simulink model "GHV_open_equation"  (R2023b)
settings: Solver=VariableStepAuto  StartTime=0.0  StopTime=10  FixedStep=0.0000001  MaxStep=0.1  RelTol=1e-3
libraries: simulink_extras x2
settings Model: SimulationMode=accelerator  Creator=Admin  LastModifiedBy=Admin

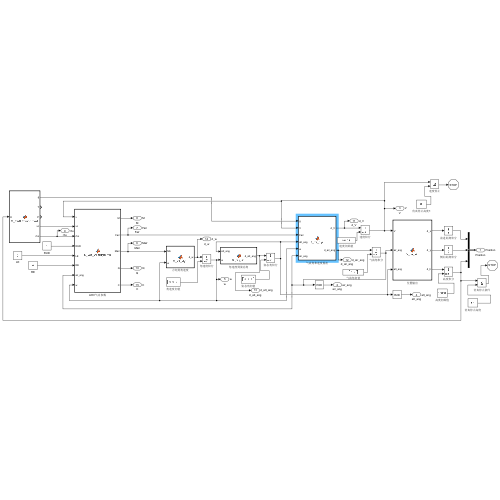
[thumbnail: Simulink's stored preview of the top-level diagram]
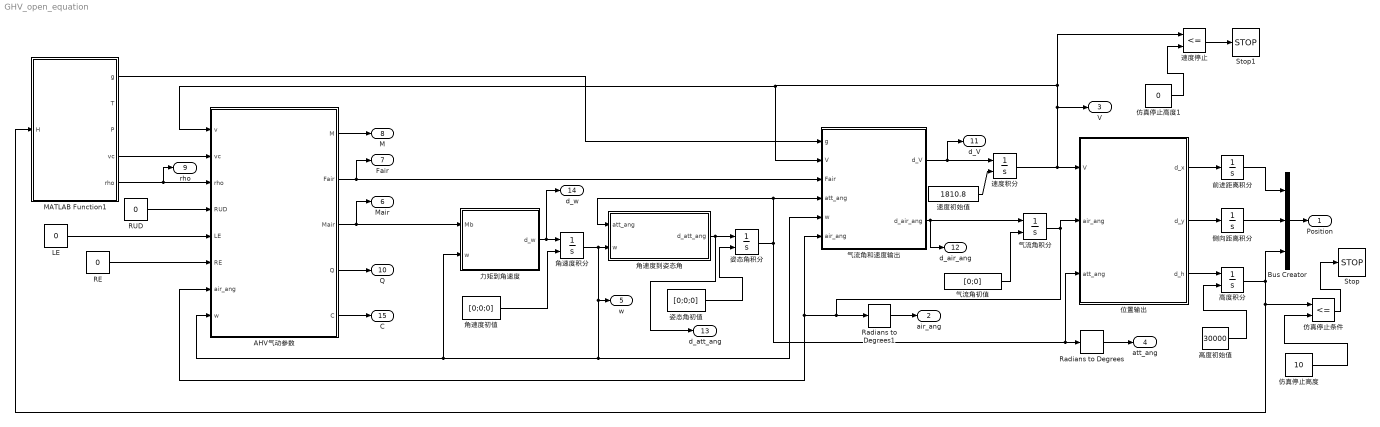
== system GHV_open_equation ==
  AHV气动参数 : MATLAB Function  TreatAsAtomicUnit=on
  Bus Creator : BusCreator  Inputs=3
  LE : Constant  Value=0
  MATLAB Function1 : MATLAB Function  TreatAsAtomicUnit=on
  RE : Constant  Value=0
  RUD : Constant  Value=0
  Radians to Degrees : simulink_extras/Transformations/Radians to Degrees
  Radians to Degrees1 : simulink_extras/Transformations/Radians to Degrees
  Stop : Stop
  Stop1 : Stop
  仿真停止条件 : RelationalOperator  Operator=<=  OutDataTypeStr=boolean  RndMeth=Simplest  InputSameDT=off
  仿真停止高度 : Constant  Value=10
  仿真停止高度1 : Constant  Value=0
  位置输出 : MATLAB Function  TreatAsAtomicUnit=on
  侧向距离积分 : Integrator
  前进距离积分 : Integrator
  力矩到角速度 : MATLAB Function  TreatAsAtomicUnit=on
  姿态角初值 : Constant  Value=[0;0;0]
  姿态角积分 : Integrator  InitialConditionSource=external  InitialCondition=[0;0;0]
  气流角初值 : Constant  Value=[0;0]
  气流角和速度输出 : MATLAB Function  TreatAsAtomicUnit=on
  气流角积分 : Integrator  InitialConditionSource=external  InitialCondition=[0;0]
  角速度初值 : Constant  Value=[0;0;0]
  角速度到姿态角 : MATLAB Function  TreatAsAtomicUnit=on
  角速度积分 : Integrator  InitialConditionSource=external  InitialCondition=[0;0;0]
  速度停止 : RelationalOperator  Operator=<=  OutDataTypeStr=boolean  RndMeth=Simplest  InputSameDT=off
  速度初始值 : Constant  Value=1810.8
  速度积分 : Integrator  InitialConditionSource=external  InitialCondition=2*340
  高度初始值 : Constant  Value=30000
  高度积分 : Integrator  InitialConditionSource=external  InitialCondition=80000
  Position : Outport  SignalName=Position
  air_ang : Outport  Port=2  SignalName=air_ang
  V : Outport  Port=3  SignalName=V
  att_ang : Outport  Port=4  SignalName=att_ang
  w : Outport  Port=5  SignalName=w
  Mair : Outport  Port=6  SignalName=Mair
  Fair : Outport  Port=7  SignalName=Fair
  M : Outport  Port=8  SignalName=M
  rho : Outport  Port=9  SignalName=rho
  Q : Outport  Port=10  SignalName=Q
  d_V : Outport  Port=11  SignalName=d_V
  d_air_ang : Outport  Port=12  SignalName=d_air_ang
  d_att_ang : Outport  Port=13  SignalName=d_att_ang
  d_w : Outport  Port=14  SignalName=d_w
  C : Outport  Port=15  SignalName=C
  wires:
  力矩到角速度/1(d_w) -> d_w/1, 角速度积分/1
  角速度积分/1 -> 气流角和速度输出/5(w), 力矩到角速度/2(w), AHV气动参数/8(w), w/1, 角速度到姿态角/2(w)
  角速度到姿态角/1(d_att_ang) -> 姿态角积分/1, d_att_ang/1
  姿态角积分/1 -> 气流角和速度输出/4(att_ang), 角速度到姿态角/1(att_ang), 位置输出/3(att_ang), Radians to Degrees/1
  气流角积分/1 -> 位置输出/2(air_ang), 气流角和速度输出/6(air_ang), AHV气动参数/7(air_ang), Radians to Degrees1/1
  气流角和速度输出/1(d_V) -> d_V/1, 速度积分/1
  AHV气动参数/2(Fair) -> 气流角和速度输出/3(Fair), Fair/1
  MATLAB Function1/5(rho) -> AHV气动参数/3(rho), rho/1
  MATLAB Function1/4(vc) -> AHV气动参数/2(vc)
  MATLAB Function1/1(g) -> 气流角和速度输出/1(g)
  位置输出/1(d_x) -> 前进距离积分/1
  位置输出/2(d_y) -> 侧向距离积分/1
  位置输出/3(d_h) -> 高度积分/1
  侧向距离积分/1 -> Bus Creator/2
  前进距离积分/1 -> Bus Creator/1
  Bus Creator/1 -> Position/1
  Radians to Degrees/1 -> att_ang/1
  Radians to Degrees1/1 -> air_ang/1
  RUD/1 -> AHV气动参数/4(RUD)
  仿真停止条件/1 -> Stop/1
  高度积分/1 -> 仿真停止条件/1, MATLAB Function1/1(H), Bus Creator/3
  AHV气动参数/1(M) -> M/1
  高度初始值/1 -> 高度积分/2
  速度初始值/1 -> 速度积分/2
  仿真停止高度/1 -> 仿真停止条件/2
  AHV气动参数/4(Q) -> Q/1
  速度积分/1 -> V/1, 速度停止/1, 气流角和速度输出/2(V), AHV气动参数/1(v), 位置输出/1(V)
  仿真停止高度1/1 -> 速度停止/2
  速度停止/1 -> Stop1/1
  气流角和速度输出/2(d_air_ang) -> 气流角积分/1, d_air_ang/1
  AHV气动参数/5(C) -> C/1
  AHV气动参数/3(Mair) -> 力矩到角速度/1(Mb), Mair/1
  RE/1 -> AHV气动参数/6(RE)
  LE/1 -> AHV气动参数/5(LE)
  角速度初值/1 -> 角速度积分/2
  姿态角初值/1 -> 姿态角积分/2
  气流角初值/1 -> 气流角积分/2

== matlab function GHV_open_equation/角速度到姿态角 ==
  data: att_ang input; w input; d_att_ang output
function d_att_ang = S_rot_kin(att_ang, w)

    d_att_ang = rot_kin(att_ang, w);

end

== matlab function GHV_open_equation/力矩到角速度 ==
  data: Mb input; d_w output; w input
function d_w  = S_rot_dyn (Mb, w)

    d_w = zeros(3, 1); %#ok<*PREALL>
    [d_w] = rot_dyn(Mb, w);


end

== matlab function GHV_open_equation/气流角和速度输出 ==
  data: g input; V input; Fair input; d_V output; att_ang input; w input; air_ang input; d_air_ang output
function [d_V, d_air_ang] = S_tra_dyn(g, V, Fair, att_ang, w, air_ang)

     d_V = zeros(1, 1);
     d_air_ang = zeros(2, 1);
    [d_V, d_air_ang] = tra_dyn(Fair, g, V, air_ang, att_ang, w);



end

== matlab function GHV_open_equation/AHV气动参数 ==
  data: M output; v input; vc input; rho input; RUD input; LE input; RE input; Fair output; air_ang input; w input; Mair output; Q output; C output
function [M, Fair, Mair, Q, C] = S_Get_Aerodynamic(v, vc, rho, RUD, LE, RE, air_ang, w)

  
[M, Fair, Mair, Q, C] = Get_Aerodynamic(LE, RE, RUD, air_ang, v, w, vc, rho);
   
end

== matlab function GHV_open_equation/MATLAB Function1 ==
  data: g output; H input; T output; P output; vc output; rho output
function [g, T, P, vc, rho] = S_EarthEnvironment(H)

[T, vc, P, rho, g] = EarthEnvironment(H);

end

== matlab function GHV_open_equation/位置输出 ==
  data: V input; d_x output; air_ang input; att_ang input; d_y output; d_h output
function [d_x, d_y, d_h] = S_tra_kin(V, air_ang, att_ang)

   [d_x, d_y, d_h] = tra_kin(V, air_ang, att_ang);

end
